simulink model "labTWOsecTWO"  (R2023b)
settings: Solver=VariableStepAuto  StartTime=0.0  StopTime=10.0  RelTol=1e-3
settings Model: Creator=omarf  LastModifiedBy=omarf

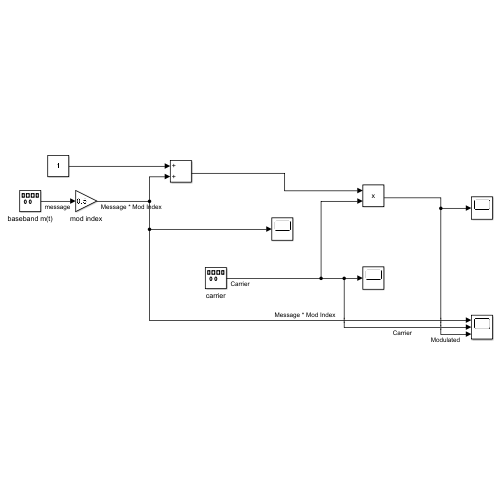
[thumbnail: Simulink's stored preview of the top-level diagram]
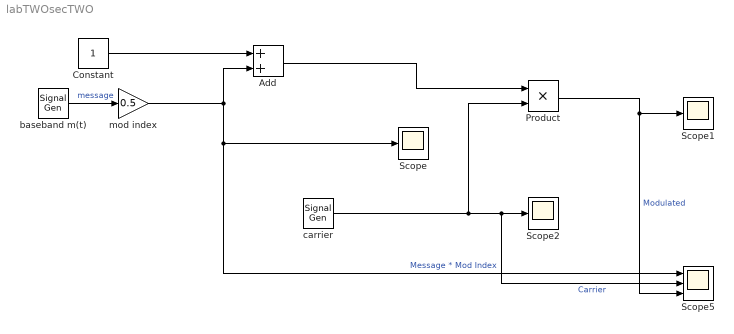
== system labTWOsecTWO ==
  Add : Sum
  Constant : Constant
  Product : Product
  Scope : Scope
  Scope1 : Scope
  Scope2 : Scope
  Scope5 : Scope  NumInputPorts=3
  baseband m(t) : SignalGenerator  Frequency=1000
  carrier : SignalGenerator  Frequency=20000
  mod index : Gain  Gain=0.5
  wires:
  baseband m(t)/1 -> mod index/1  "message"
  Product/1 -> Scope5/3, Scope1/1  "Modulated"
  carrier/1 -> Scope5/2, Scope2/1, Product/2  "Carrier"
  mod index/1 -> Add/2, Scope5/1, Scope/1  "Message * Mod Index"
  Constant/1 -> Add/1
  Add/1 -> Product/1
